simulink model "Anti_Surge_Controller_Revised"  (R2021a)
settings: Solver=VariableStepAuto  StartTime=0.0  StopTime=100  RelTol=1e-3
values from neighbouring files (symbols this model uses):
  AolT = sys_dt.A    [zhu_model_magnetic_bearing.m]
  BolT = sys_dt.B    [zhu_model_magnetic_bearing.m]
  c = c1+c2+c3+c4+c5+c6    [zhu_model_magnetic_bearing.m]
  ColT = sys_dt.C    [zhu_model_magnetic_bearing.m]
  DolT = sys_dt.D    [zhu_model_magnetic_bearing.m]
  k = 25    [zhu_model_magnetic_bearing.m]
  Ki = Kflux*N/Ro    [zhu_model_magnetic_bearing.m]
  Kx = Kflux^2/Ro/25000    [zhu_model_magnetic_bearing.m]
  m = 330    [zhu_model_magnetic_bearing.m]
  P0T = 10^-3    (= 0.001)    [zhu_model_magnetic_bearing.m]
  QcovT = 10^-5    (= 1e-05)    [zhu_model_magnetic_bearing.m]
  RcovT = 10^-4    (= 0.0001)    [zhu_model_magnetic_bearing.m]
  s = fotf('s')    [zhu_model_magnetic_bearing.m]
  x0T = 0    [zhu_model_magnetic_bearing.m]
undefined symbols (not defined in the file or in its folder): K1, K2, P0, Qcov, Rcov, sys_d, x0c
libraries: simulink x4, fod x2
settings Model: Creator=NATO  LastModifiedBy=macbookpro
settings SolverCC: AlgebraicLoopSolver=TrustRegion
settings DataIOCC: ReturnWorkspaceOutputs=off
settings DebuggingCC: SFMachineParentedDataDiag=warning  ArithmeticOperatorsInVariantConditions=warning
settings SFSimCC: SimUseLocalCustomCode=off  CustomCodeUndefinedFunction=UseInterfaceOnly
settings RTWCC: RTWUseLocalCustomCode=off
settings CodeAppCC: StateflowObjectComments=on

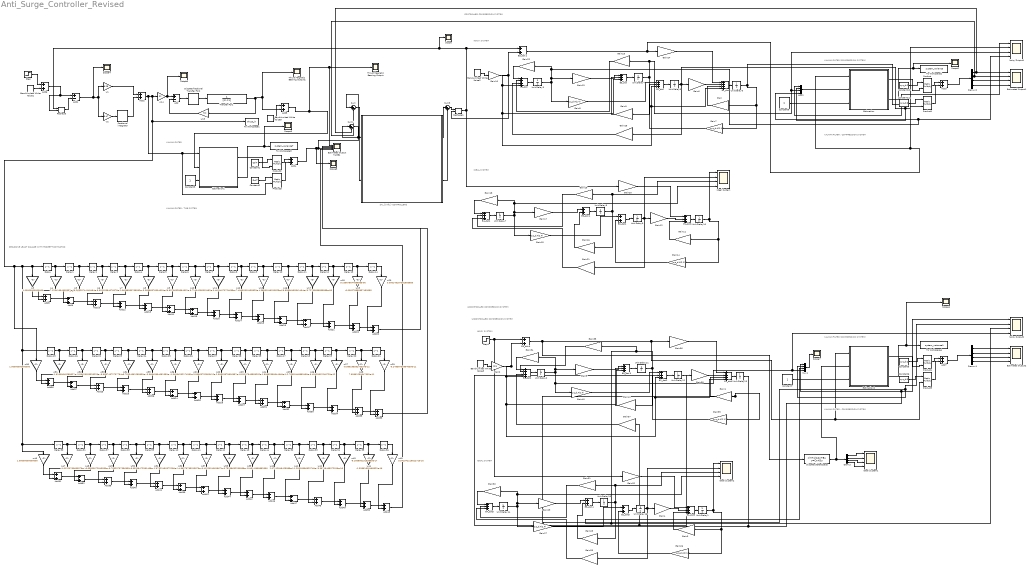
== system Anti_Surge_Controller_Revised ==
  note: RECURSIVE LEAST SQUARE WITH FORGETTING FACTOR
  note: KALMAN FILTER (COMPRESSION SYSTEM)
  note: IDEAL SYSTEM
  note: NOISY SYSTEM
  note: KALMAN FILTER
  note: NOISY SYSTEM
  note: IDEAL SYSTEM
  note: KALMAN FILTER (COMPRESSION SYSTEM)
  note: CONTROLLED COMPRESSION SYSTEM
  note: UNCONTROLLED COMPRESSION SYSTEM
  note: KALMAN FILTER : TMB SYSTEM
  note: KALMAN FILTER : COMPRESSION SYSTEM
  note: KALMAN FILTER : COMPRESSION SYSTEM
  note: $H_{\infty} CONTROLLER$
  note: UNCONTROLLED COMPRESSION SYSTEM
  " " : Subsystem
  Add : Sum  Inputs=+-
  Add1 : Sum  Inputs=+-
  Add{2..52} (51 alike) : Sum
  Band-Limited White Noise1 : simulink/Sources/Band-Limited White Noise  Cov=[10^-10]  Ts=1  seed=[23341]
  Band-Limited White Noise2 : simulink/Sources/Band-Limited White Noise  Cov=[1]  Ts=0.05  seed=[23341]
  Band-Limited White Noise3 : simulink/Sources/Band-Limited White Noise  Cov=[1]  Ts=0.005  seed=[23341]
  Band-Limited White Noise5 : simulink/Sources/Band-Limited White Noise  Cov=[10^-8]  Ts=0.1  seed=[23341]
  Constant1 : Constant  Value=ColT  VectorParams1D=off
  Constant10 : Constant  Value=sys_d.C  VectorParams1D=off
  Constant11 : Constant  Value=sys_d.D  VectorParams1D=off
  Constant2 : Constant  Value=DolT  VectorParams1D=off
  Constant3 : Constant  VectorParams1D=off
  Constant5 : Constant  Value=sys_d.C  VectorParams1D=off
  Constant6 : Constant  Value=sys_d.D  VectorParams1D=off
  Constant7 : Constant  VectorParams1D=off
  Constant9 : Constant  VectorParams1D=off
  Delay{,1..44} (45 alike) : Delay  DelayLength=1  InitialCondition=0
  Demux : Demux
  Demux1 : Demux
  Demux2 : Demux
  Discrete State-Space : DiscreteStateSpace  A=sys_d.A  B=sys_d.B  C=sys_d.C  D=sys_d.D  SampleTime=0.005
  Discrete fractional Transfer Fcn2 : fod/Discrete fractional Transfer Fcn  zeroPoly=53900  polePoly=53900+10432*s^0.5  freqRange=[0.001, 10000]  approxNum=5  useRef=off  dscrMethod=Matched  wc=0  ts=0.1
      settings: SourceProductName=FOMCON Toolbox
  E1_dot : Sum  Inputs=++++
  E1_dot1 : Sum  Inputs=+++
  E1_dot2 : Sum  Inputs=++++
  E1_dot3 : Sum  Inputs=+++
  E2_dot : Sum  Inputs=+++
  E2_dot1 : Sum
  E2_dot2 : Sum  Inputs=+++
  E2_dot3 : Sum
  "E3_dot " : Sum  Inputs=+++
  E3_dot {1..2,4..5} (4 alike) : Sum
  E3_dot 3 : Sum  Inputs=+++
  E4_dot : Sum  Inputs=++++
  E4_dot1 : Sum  Inputs=+++
  E4_dot2 : Sum  Inputs=++++
  E4_dot3 : Sum  Inputs=+++
  Estimated Output TAMB1 : Scope  NumInputPorts=5
  Estimated Output1 : Scope  NumInputPorts=4
  Estimated Output2 : Scope  NumInputPorts=4
  Estimation : Subsystem
  Estimation1 : Subsystem
  Estimation2 : Subsystem
  Fractional integrator : fod/Fractional integrator  gam=0.5  ww=[0.001; 1000]  n=5  nFod=off
      settings: SourceProductName=FOMCON Toolbox
  Gain{,1,3,11} (4 alike) : Gain  Gain=sys_d.A(1,1)
  Gain10 : Gain  Gain=0.00001
  Gain{4,6,12,38} (4 alike) : Gain  Gain=sys_d.A(1,2)
  Gain{5,13,17,19,23,29,31,35} (8 alike) : Gain  Gain=sys_d.A(3,4)
  Gain{7,14,26,39} (4 alike) : Gain  Gain=sys_d.A(2,1)
  Gain{8,15,21,25,27,33,37,40} (8 alike) : Gain  Gain=sys_d.A(2,4)
  Gain{9,16,28,41} (4 alike) : Gain  Gain=sys_d.A(3,3)
  Gain{18,22,30,34} (4 alike) : Gain  Gain=sys_d.A(4,4)
  Gain2 : Gain  Gain=0.1
  Gain{20,24,32,36} (4 alike) : Gain  Gain=sys_d.B(1,1)
  Ideal System : Scope  NumInputPorts=4
  Ideal System1 : Scope  NumInputPorts=4
  Ideal System2 : Scope  NumInputPorts=4
  Mux1 : Mux
  Mux2 : Mux
  Noisy Output1 : Scope  NumInputPorts=4
  Noisy Output2 : Scope  NumInputPorts=4
  Product{,1..5} (6 alike) : Product  Multiplication=Matrix(*)
  Reshape : Reshape  OutputDimensionality=Derive from reference input port
  Reshape1 : Reshape  OutputDimensionality=Derive from reference input port
  Scope{,1..7} (8 alike) : Scope
  Step : Step  After=1.5*10^-4  SampleTime=0
  Step1 : Step  SampleTime=0.005
  Sum : Sum  Inputs=|+-
  Sum1 : Sum  Inputs=|+-
  Sum3 : Sum  Inputs=|++
  Thrust Magnetic Bearing Output : Scope
  Thrust Magnetic Bearing Output1 : Scope
  To Workspace1 : ToWorkspace  VariableName=thrust_in  SampleTime=0.1
      settings: Save2DSignal=2-D array (concatenate along first dimension)
  To Workspace2 : ToWorkspace  VariableName=system_variance  SampleTime=-1
      settings: MaxDataPoints=1
  To Workspace3 : ToWorkspace  VariableName=system_varianceT  SampleTime=-1
      settings: MaxDataPoints=1
  To Workspace4 : ToWorkspace  VariableName=system_variance1  SampleTime=-1
      settings: MaxDataPoints=1
  Transfer Fcn1 : TransferFcn  Denominator=[m c k]
  Unit Delay{1..2,11..16} (8 alike) : UnitDelay  SampleTime=0.005  HasFrameUpgradeWarning=on
  Unit Delay{3..10} (8 alike) : UnitDelay  SampleTime=-1  HasFrameUpgradeWarning=on
  w1 : Gain  Gain=9.25
  w10 : Gain  Gain=5.71434208313482e-06
  w11 : Gain  Gain=5.44314070724695e-06
  w12 : Gain  Gain=7.49630310435823e-06
  w13 : Gain  Gain=4.36661046310525e-05
  w14 : Gain  Gain=Ki
  w15 : Gain  Gain=Kx
  w16 : Gain  Gain=8.89806493541494e-06
  w17 : Gain  Gain=5.72750856859985e-06
  w18 : Gain  Gain=9.10967864788686e-06
  w19 : Gain  Gain=-0.000278855937453055
  w2 : Gain  Gain=3.47
  w20 : Gain  Gain=0.000145187092666685
  w21 : Gain  Gain=3.05363732083412e-13
  w22 : Gain  Gain=2.90813879816957e-12
  w23 : Gain  Gain=8.81147845559202e-12
  w24 : Gain  Gain=1.80692390644948e-12
  w25 : Gain  Gain=-2.70615448883499e-11
  w26 : Gain  Gain=6.45429512248729e-12
  w27 : Gain  Gain=-5.95929555270337e-12
  w28 : Gain  Gain=7.69961250647502e-11
  w29 : Gain  Gain=-6.24538793994039e-11
  w3 : Gain  Gain=1.00000000000000
  w30 : Gain  Gain=1.00000000000000
  w31 : Gain  Gain=-1.61509045285627e-11
  w32 : Gain  Gain=3.55425153326229e-12
  w33 : Gain  Gain=-8.68574372797784e-12
  w34 : Gain  Gain=5.79134561289939e-11
  w35 : Gain  Gain=-3.96643994081353e-11
  w36 : Gain  Gain=-1.54354252174381e-12
  w37 : Gain  Gain=-3.41220240818674e-16
  w38 : Gain  Gain=5.75138632250958e-17
  w39 : Gain  Gain=10431.8999882690
  w4 : Gain  Gain=7.12541994903337e-06
  w40 : Gain  Gain=2.07112848425985e-16
  w41 : Gain  Gain=1.29318596823748e-16
  w42 : Gain  Gain=5.38716465372916e-16
  w43 : Gain  Gain=-8.16080013153855e-17
  w44 : Gain  Gain=-1.33861815468522e-16
  w45 : Gain  Gain=5.54154221662272e-16
  w46 : Gain  Gain=1.00000000000000
  w47 : Gain  Gain=-1.01120760660376e-16
  w48 : Gain  Gain=-6.63600072843550e-18
  w49 : Gain  Gain=-9.70523797356939e-16
  w5 : Gain  Gain=6.26329744149484e-06
  w50 : Gain  Gain=8.90108472381468e-17
  w51 : Gain  Gain=1.67922450372206e-16
  w52 : Gain  Gain=-4.86276795313876e-16
  w6 : Gain  Gain=5.93115384076078e-06
  w7 : Gain  Gain=2.64598950768992e-06
  w8 : Gain  Gain=5.08988376604610e-06
  w9 : Gain  Gain=6.83706528664812e-06
  wires:
  Transfer Fcn1/1 -> Thrust Magnetic Bearing Output1/1, Add5/2, w15/1
  w15/1 -> Add/2
  Add/1 -> Discrete fractional Transfer Fcn2/1
  Add1/1 -> Scope4/1, w1/1, w2/1
  w14/1 -> Scope6/1, Add/1
  Discrete fractional Transfer Fcn2/1 -> Transfer Fcn1/1
  Band-Limited White Noise5/1 -> Add5/1
  Sum/1 -> " "/2(In1)
  Demux2/1 -> Estimated Output1/1, Sum1/2
  Demux2/2 -> Estimated Output1/2, Sum/2
  w1/1 -> Add2/1
  w2/1 -> Fractional integrator/1
  Fractional integrator/1 -> Add2/2
  Add4/1 -> Scope5/1, Sum/1, Sum1/1, Estimated Output TAMB1/4  "Kalman Filter"
  Gain16/1 -> E3_dot 1/2
  Constant10/1 -> Product/1
  E4_dot/1 -> Unit Delay3/1
  Unit Delay9/1 -> Ideal System/2, Gain12/1, Gain21/1  "E2"
  Gain25/1 -> E4_dot/3
  Gain/1 -> E1_dot/3
  Gain24/1 -> E1_dot/1  "input"
  Gain13/1 -> "E3_dot "/1
  Gain8/1 -> E2_dot/1
  E2_dot/1 -> Unit Delay5/1
  Gain23/1 -> E4_dot/2
  Unit Delay5/1 -> Mux2/2, Noisy Output1/2, Gain6/1, Gain25/1  "E2"
  Gain20/1 -> E1_dot1/1  "input"
  Constant9/1 -> Estimation/3(Active)
  Unit Delay6/1 -> Gain7/1, Gain/1, Mux2/1, Noisy Output1/1  "E1"
  Product1/1 -> Add3/2
  Estimation/2(Out2) -> Scope2/1, To Workspace2/1
  Gain6/1 -> E1_dot/2
  Add3/1 -> Demux2/1
  Gain7/1 -> E2_dot/2
  Constant11/1 -> Product1/1
  E1_dot1/1 -> Unit Delay10/1
  Demux2/3 -> Estimated Output1/3
  Demux2/4 -> Estimated Output1/4
  Gain18/1 -> E4_dot1/1
  "E3_dot "/1 -> Unit Delay4/1
  Gain10/1 -> Reshape1/2, E4_dot/4, E1_dot/4, E2_dot/3, "E3_dot "/3, E3_dot 2/2
  E2_dot1/1 -> Unit Delay9/1
  Gain11/1 -> E1_dot1/3
  Gain9/1 -> "E3_dot "/2
  Unit Delay3/1 -> Gain22/1, Noisy Output1/4, Mux2/4, Gain13/1, Gain8/1  "E4"
  Mux2/1 -> Estimation/2(y[k])
  Gain17/1 -> E3_dot 1/1
  Unit Delay7/1 -> Gain18/1, Ideal System/4, Gain17/1, Gain15/1  "E4"
  Unit Delay10/1 -> Gain14/1, Gain11/1, Ideal System/1  "E1"
  Product/1 -> Add3/1
  Gain12/1 -> E1_dot1/2
  E4_dot1/1 -> Unit Delay7/1
  Estimation/1(x̂[k|k]) -> Product/2
  E1_dot/1 -> Unit Delay6/1
  Unit Delay4/1 -> Gain9/1, Gain23/1, Noisy Output1/3, Mux2/3  "E3"
  Unit Delay8/1 -> Gain16/1, Gain19/1, Ideal System/3  "E3"
  E3_dot 1/1 -> Unit Delay8/1
  Gain15/1 -> E2_dot1/1
  Gain19/1 -> E4_dot1/2
  Gain22/1 -> E4_dot/1
  Gain21/1 -> E4_dot1/3
  Gain14/1 -> E2_dot1/2
  Band-Limited White Noise2/1 -> Gain10/1
  E3_dot 2/1 -> Gain24/1, Product1/2, Estimation/1(u[k])
  Sum1/1 -> " "/1(In2)
  Reshape1/1 -> Gain20/1, Reshape/1, Scope/1, E3_dot 2/1
  Product2/1 -> Add4/1
  Constant3/1 -> Estimation1/3(Active)
  Product3/1 -> Add4/2
  Constant2/1 -> Product3/1
  Constant1/1 -> Product2/1
  Add2/1 -> Product3/2, Estimation1/1(u[k]), Delay15/1, Delay30/1, w46/1, Delay/1, w3/1, w30/1, To Workspace1/1, w14/1
  Add5/1 -> Estimation1/2(y[k]), Thrust Magnetic Bearing Output/1, Estimated Output TAMB1/1  "Real Output TMB"
  Estimation1/1(x̂[k|k]) -> Product2/2
  Estimation1/2(Out2) -> Scope3/1, To Workspace3/1
  Band-Limited White Noise1/1 -> Add6/2
  Step/1 -> Add6/1
  Constant6/1 -> Product5/1
  Gain2/1 -> E3_dot 5/2, E4_dot2/4, E1_dot2/4, E2_dot2/3, E3_dot 3/3
  Gain35/1 -> E4_dot2/2
  E3_dot 3/1 -> Unit Delay11/1
  E3_dot 5/1 -> Discrete State-Space/1, Product5/2, Estimation2/1(u[k]), Gain36/1
  E1_dot2/1 -> Unit Delay13/1
  Demux1/2 -> Estimated Output2/2
  Gain31/1 -> E4_dot3/2
  E4_dot3/1 -> Unit Delay14/1
  Constant7/1 -> Estimation2/3(Active)
  Gain36/1 -> E1_dot2/1  "input"
  Gain37/1 -> E4_dot2/3
  Gain1/1 -> E1_dot2/3
  Gain3/1 -> E1_dot3/3
  Unit Delay14/1 -> Gain30/1, Ideal System2/4, Gain29/1, Gain27/1  "E4"
  Gain4/1 -> E1_dot3/2
  E2_dot3/1 -> Unit Delay16/1
  Gain28/1 -> E3_dot 4/2
  Constant5/1 -> Product4/1
  Unit Delay16/1 -> Ideal System2/2, Gain4/1, Gain33/1  "E2"
  Demux1/4 -> Estimated Output2/4
  Gain32/1 -> E1_dot3/1  "input"
  Product4/1 -> Add7/1
  Gain40/1 -> E2_dot2/1
  E1_dot3/1 -> Unit Delay1/1
  Gain27/1 -> E2_dot3/1
  Gain38/1 -> E1_dot2/2
  Gain34/1 -> E4_dot2/1
  E3_dot 4/1 -> Unit Delay15/1
  Unit Delay12/1 -> Gain38/1, Noisy Output2/2, Mux1/2, Gain37/1  "E2"
  Unit Delay13/1 -> Gain39/1, Gain1/1, Noisy Output2/1, Mux1/1  "E1"
  Demux1/3 -> Estimated Output2/3
  Gain30/1 -> E4_dot3/1
  Product5/1 -> Add7/2
  Gain41/1 -> E3_dot 3/2
  Gain39/1 -> E2_dot2/2
  Unit Delay15/1 -> Gain28/1, Gain31/1, Ideal System2/3  "E3"
  Gain29/1 -> E3_dot 4/1
  Unit Delay2/1 -> Noisy Output2/4, Mux1/4, Gain40/1, Gain34/1, Gain5/1  "E4"
  Unit Delay11/1 -> Gain41/1, Gain35/1, Mux1/3, Noisy Output2/3  "E3"
  Unit Delay1/1 -> Gain26/1, Gain3/1, Ideal System2/1  "E1"
  E2_dot2/1 -> Unit Delay12/1
  Gain5/1 -> E3_dot 3/1
  Gain33/1 -> E4_dot3/3
  Add7/1 -> Demux1/1
  Gain26/1 -> E2_dot3/2
  Band-Limited White Noise3/1 -> Gain2/1
  Estimation2/1(x̂[k|k]) -> Product4/2
  Estimation2/2(Out2) -> Scope1/1, To Workspace4/1
  E4_dot2/1 -> Unit Delay2/1
  Demux1/1 -> Estimated Output2/1
  " "/1(Out1) -> Sum3/1
  " "/2(Out2) -> Sum3/2
  Delay1/1 -> Delay2/1, w5/1
  Delay/1 -> Delay1/1, w4/1
  w3/1 -> Add8/1
  w4/1 -> Add8/2
  Add8/1 -> Add9/1
  w5/1 -> Add9/2
  Delay2/1 -> Delay3/1, w6/1
  w6/1 -> Add10/2
  Add9/1 -> Add10/1
  Delay3/1 -> w7/1, Delay4/1
  Delay4/1 -> w8/1, Delay5/1
  Delay5/1 -> w9/1, Delay6/1
  Delay6/1 -> w10/1, Delay7/1
  Delay7/1 -> Delay8/1, w11/1
  Delay8/1 -> Delay9/1, w12/1
  Delay9/1 -> Delay10/1, w13/1
  Delay10/1 -> Delay11/1, w16/1
  Delay11/1 -> Delay12/1, w17/1
  Delay12/1 -> Delay13/1, w18/1
  Delay13/1 -> Delay14/1, w19/1
  Add13/1 -> Add11/1
  Add6/1 -> Add1/1, Reshape/2
  Add12/1 -> Add13/1
  Add15/1 -> Add16/1
  Add16/1 -> Add14/1
  Add10/1 -> Add12/1
  w7/1 -> Add12/2
  w8/1 -> Add13/2
  w9/1 -> Add11/2
  Add11/1 -> Add15/1
  w10/1 -> Add15/2
  w11/1 -> Add16/2
  Delay14/1 -> w20/1
  w12/1 -> Add14/2
  Add18/1 -> Add19/1
  w17/1 -> Add17/2
  w16/1 -> Add19/2
  Add19/1 -> Add17/1
  Add22/1 -> Add20/1
  w20/1 -> Add20/2
  w19/1 -> Add22/2
  Add21/1 -> Add22/1
  Add14/1 -> Add18/1  "RLS : Lambda =1"
  w13/1 -> Add18/2
  Add17/1 -> Add21/1  "RLS : Lambda =1"
  w18/1 -> Add21/2
  Add20/1 -> Estimated Output TAMB1/2  "RLS : Lambda =1"
  Delay16/1 -> Delay22/1, w32/1
  w36/1 -> Add24/2
  Add26/1 -> Add24/1
  w30/1 -> Add36/1
  w31/1 -> Add36/2
  Add23/1 -> Add25/1
  Add36/1 -> Add37/1
  Add28/1 -> Add29/1
  Delay15/1 -> Delay16/1, w31/1
  w26/1 -> Add30/2
  Delay22/1 -> Delay23/1, w33/1
  w25/1 -> Add32/2
  w33/1 -> Add23/2
  Delay27/1 -> Delay28/1, w22/1
  w29/1 -> Add33/2
  w35/1 -> Add26/2
  Delay23/1 -> w34/1, Delay24/1
  w32/1 -> Add37/2
  Add34/1 -> Add35/1
  Delay21/1 -> w29/1
  Delay25/1 -> w36/1, Delay26/1
  Add29/1 -> Add27/1
  Delay20/1 -> Delay21/1, w28/1
  Delay19/1 -> Delay20/1, w27/1
  Delay24/1 -> w35/1, Delay25/1
  w22/1 -> Add29/2
  w24/1 -> Add31/2
  Add25/1 -> Add26/1
  Add37/1 -> Add23/1
  w28/1 -> Add35/2
  Delay28/1 -> Delay29/1, w23/1
  Add30/1 -> Add34/1  "RLS : Lambda =1"
  w21/1 -> Add28/2
  Add27/1 -> Add31/1  "RLS : Lambda =1"
  Add32/1 -> Add30/1
  Add31/1 -> Add32/1
  w34/1 -> Add25/2
  Delay17/1 -> Delay18/1, w25/1
  Add24/1 -> Add28/1
  w27/1 -> Add34/2
  Add35/1 -> Add33/1
  Delay26/1 -> w21/1, Delay27/1
  Delay29/1 -> Delay17/1, w24/1
  w23/1 -> Add27/2
  Delay18/1 -> Delay19/1, w26/1
  Delay31/1 -> Delay37/1, w48/1
  w52/1 -> Add39/2
  Add41/1 -> Add39/1
  w46/1 -> Add51/1
  w47/1 -> Add51/2
  Add38/1 -> Add40/1
  Add51/1 -> Add52/1
  Add43/1 -> Add44/1
  Delay30/1 -> Delay31/1, w47/1
  w42/1 -> Add45/2
  Delay37/1 -> Delay38/1, w49/1
  w41/1 -> Add47/2
  w49/1 -> Add38/2
  Delay42/1 -> Delay43/1, w38/1
  w45/1 -> Add48/2
  w51/1 -> Add41/2
  Delay38/1 -> w50/1, Delay39/1
  w48/1 -> Add52/2
  Add49/1 -> Add50/1
  Delay36/1 -> w45/1
  Delay40/1 -> w52/1, Delay41/1
  Add44/1 -> Add42/1
  Delay35/1 -> Delay36/1, w44/1
  Delay34/1 -> Delay35/1, w43/1
  Delay39/1 -> w51/1, Delay40/1
  w38/1 -> Add44/2
  w40/1 -> Add46/2
  Add40/1 -> Add41/1
  Add52/1 -> Add38/1
  w44/1 -> Add50/2
  Delay43/1 -> Delay44/1, w39/1
  Add45/1 -> Add49/1  "RLS : Lambda =1"
  w37/1 -> Add43/2
  Add42/1 -> Add46/1  "RLS : Lambda =1"
  Add47/1 -> Add45/1
  Add46/1 -> Add47/1
  w50/1 -> Add40/2
  Delay32/1 -> Delay33/1, w41/1
  Add39/1 -> Add43/1
  w43/1 -> Add49/2
  Add50/1 -> Add48/1
  Delay41/1 -> w37/1, Delay42/1
  Delay44/1 -> Delay32/1, w40/1
  w39/1 -> Add42/2
  Delay33/1 -> Delay34/1, w42/1
  Add33/1 -> Estimated Output TAMB1/3  "RLS : Lambda =0.975"
  Add48/1 -> Estimated Output TAMB1/5  "RLS : Lambda =0.95"
  Step1/1 -> E3_dot 5/1, Gain32/1
  Discrete State-Space/1 -> Estimation2/2(y[k]), Demux/1
  Demux/1 -> Ideal System1/1
  Demux/2 -> Ideal System1/2
  Demux/3 -> Ideal System1/3
  Demux/4 -> Ideal System1/4
  Reshape/1 -> Add1/2
  Sum3/1 -> Reshape1/1
  Mux1/1 -> Scope7/1

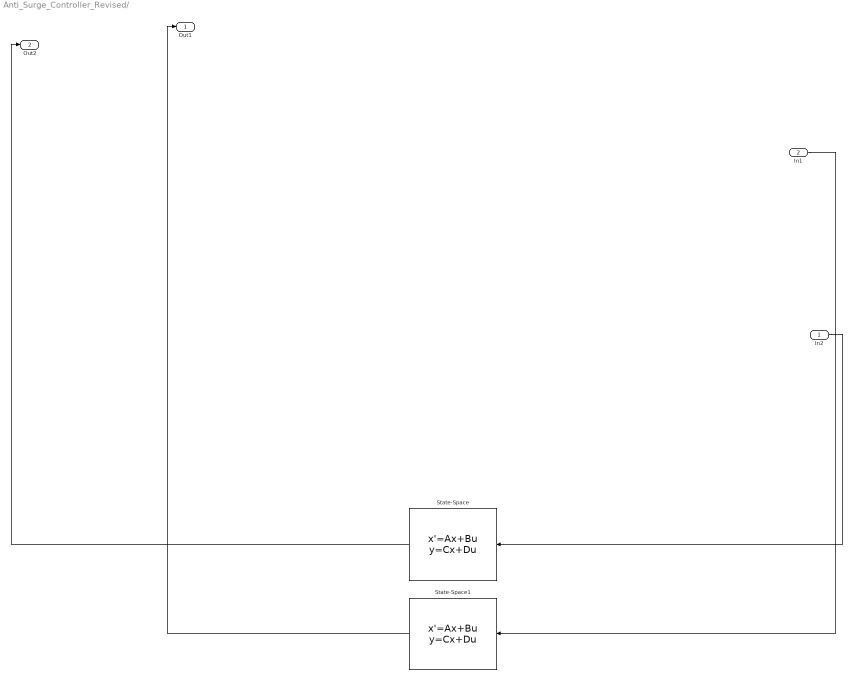
== system Anti_Surge_Controller_Revised/  ==
  In2 : Inport
  In1 : Inport  Port=2
  State-Space : StateSpace  A=K2.A  B=K2.B  C=K2.C  D=K2.D  InitialCondition=0
  State-Space1 : StateSpace  A=K1.A  B=K1.B  C=K1.C  D=K1.D  InitialCondition=0
  Out1 : Outport
  Out2 : Outport  Port=2
  wires:
  In1/1 -> State-Space1/1
  In2/1 -> State-Space/1
  State-Space1/1 -> Out1/1
  State-Space/1 -> Out2/1

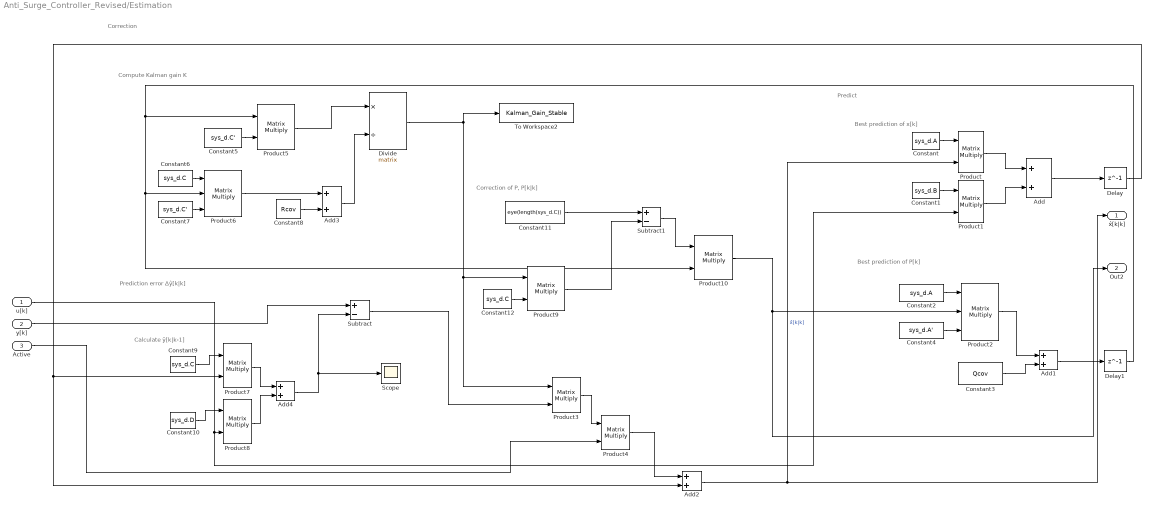
== system Anti_Surge_Controller_Revised/Estimation ==
  note: Best prediction of x[k]
  note: Predict
  note: Best prediction of P[k]
  note: Correction of P, P[k|k]
  note: Prediction error Δŷ[k|k]
  note: Compute Kalman gain K
  note: Correction
  note: Calculate ŷ[k|k-1]
  u[k] : Inport
  y[k] : Inport  Port=2
  Active : Inport  Port=3
  Add{,1..4} (5 alike) : Sum
  Constant : Constant  Value=sys_d.A  VectorParams1D=off
  Constant1 : Constant  Value=sys_d.B  VectorParams1D=off
  Constant10 : Constant  Value=sys_d.D  VectorParams1D=off
  Constant11 : Constant  Value=eye(length(sys_d.C))  VectorParams1D=off
  Constant12 : Constant  Value=sys_d.C  VectorParams1D=off
  Constant2 : Constant  Value=sys_d.A  VectorParams1D=off
  Constant3 : Constant  Value=Qcov  VectorParams1D=off
  Constant4 : Constant  Value=sys_d.A'  VectorParams1D=off
  Constant5 : Constant  Value=sys_d.C'  VectorParams1D=off
  Constant6 : Constant  Value=sys_d.C  VectorParams1D=off
  Constant7 : Constant  Value=sys_d.C'  VectorParams1D=off
  Constant8 : Constant  Value=Rcov  VectorParams1D=off
  Constant9 : Constant  Value=sys_d.C  VectorParams1D=off
  Delay : Delay  DelayLength=1  InitialCondition=x0c
  Delay1 : Delay  DelayLength=1  InitialCondition=P0
  Divide : Product  Inputs=*/  Multiplication=Matrix(*)
  Product{,1,3..5,7..10} (9 alike) : Product  Multiplication=Matrix(*)
  Product2 : Product  Inputs=3  Multiplication=Matrix(*)
  Product6 : Product  Inputs=3  Multiplication=Matrix(*)
  Scope : Scope
  Subtract : Sum  Inputs=+-
  Subtract1 : Sum  Inputs=+-
  To Workspace2 : ToWorkspace  VariableName=Kalman_Gain_Stable  SampleTime=-1
      settings: MaxDataPoints=1
  x̂[k|k] : Outport
  Out2 : Outport  Port=2
  wires:
  Constant4/1 -> Product2/3
  Constant/1 -> Product/1
  Product1/1 -> Add/2
  Constant11/1 -> Subtract1/1
  Constant6/1 -> Product6/1
  Constant12/1 -> Product9/2
  Constant2/1 -> Product2/1
  Constant3/1 -> Add1/2
  Product9/1 -> Subtract1/2
  Constant9/1 -> Product7/1
  Constant8/1 -> Add3/2
  Add3/1 -> Divide/2
  Product3/1 -> Product4/1
  u[k]/1 -> Product8/2, Product1/2
  Add/1 -> Delay/1
  Product8/1 -> Add4/2
  Add4/1 -> Subtract/2, Scope/1
  Constant5/1 -> Product5/2
  Delay/1 -> Add2/2, Product7/2
  Add2/1 -> Product/2, x̂[k|k]/1  "x̂[k|k]"
  Constant1/1 -> Product1/1
  Product/1 -> Add/1
  Active/1 -> Product4/2
  Subtract/1 -> Product3/2
  Add1/1 -> Delay1/1
  Product2/1 -> Add1/1
  Constant7/1 -> Product6/3
  Product4/1 -> Add2/1
  Delay1/1 -> Product6/2, Product10/2, Product5/1
  Product6/1 -> Add3/1
  Divide/1 -> Product3/1, Product9/1, To Workspace2/1
  y[k]/1 -> Subtract/1
  Product5/1 -> Divide/1
  Constant10/1 -> Product8/1
  Product7/1 -> Add4/1
  Product10/1 -> Out2/1, Product2/2
  Subtract1/1 -> Product10/1

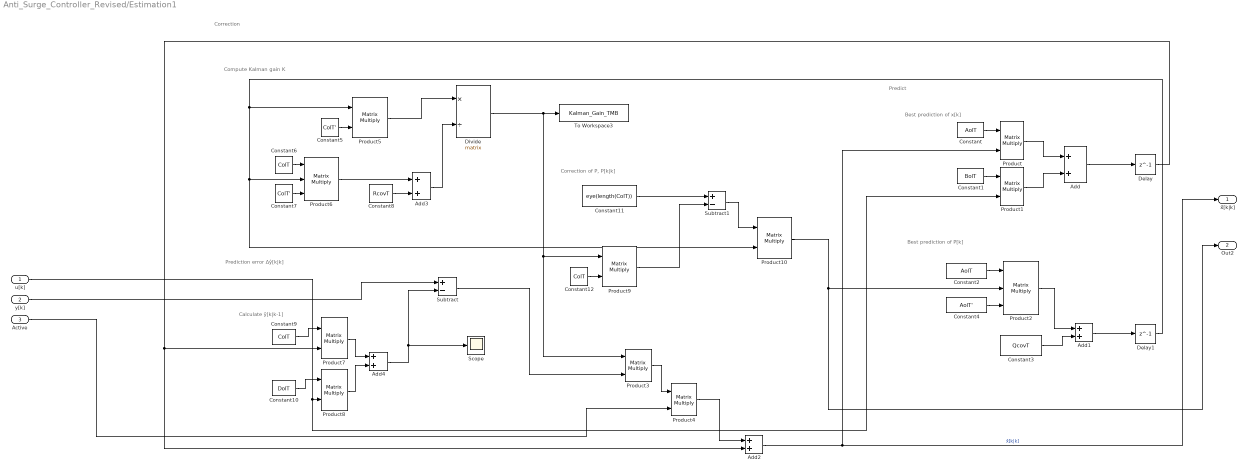
== system Anti_Surge_Controller_Revised/Estimation1 ==
  note: Best prediction of x[k]
  note: Predict
  note: Best prediction of P[k]
  note: Correction of P, P[k|k]
  note: Prediction error Δŷ[k|k]
  note: Compute Kalman gain K
  note: Correction
  note: Calculate ŷ[k|k-1]
  u[k] : Inport
  y[k] : Inport  Port=2
  Active : Inport  Port=3
  Add{,1..4} (5 alike) : Sum
  Constant : Constant  Value=AolT  VectorParams1D=off
  Constant1 : Constant  Value=BolT  VectorParams1D=off
  Constant10 : Constant  Value=DolT  VectorParams1D=off
  Constant11 : Constant  Value=eye(length(ColT))  VectorParams1D=off
  Constant12 : Constant  Value=ColT  VectorParams1D=off
  Constant2 : Constant  Value=AolT  VectorParams1D=off
  Constant3 : Constant  Value=QcovT  VectorParams1D=off
  Constant4 : Constant  Value=AolT'  VectorParams1D=off
  Constant5 : Constant  Value=ColT'  VectorParams1D=off
  Constant6 : Constant  Value=ColT  VectorParams1D=off
  Constant7 : Constant  Value=ColT'  VectorParams1D=off
  Constant8 : Constant  Value=RcovT  VectorParams1D=off
  Constant9 : Constant  Value=ColT  VectorParams1D=off
  Delay : Delay  DelayLength=1  InitialCondition=x0T
  Delay1 : Delay  DelayLength=1  InitialCondition=P0T
  Divide : Product  Inputs=*/  Multiplication=Matrix(*)
  Product{,1,3..5,7..10} (9 alike) : Product  Multiplication=Matrix(*)
  Product2 : Product  Inputs=3  Multiplication=Matrix(*)
  Product6 : Product  Inputs=3  Multiplication=Matrix(*)
  Scope : Scope
  Subtract : Sum  Inputs=+-
  Subtract1 : Sum  Inputs=+-
  To Workspace3 : ToWorkspace  VariableName=Kalman_Gain_TMB  SampleTime=-1
      settings: MaxDataPoints=1
  x̂[k|k] : Outport
  Out2 : Outport  Port=2
  wires:
  Constant4/1 -> Product2/3
  Constant/1 -> Product/1
  Product1/1 -> Add/2
  Constant11/1 -> Subtract1/1
  Constant6/1 -> Product6/1
  Constant12/1 -> Product9/2
  Constant2/1 -> Product2/1
  Constant3/1 -> Add1/2
  Product9/1 -> Subtract1/2
  Constant9/1 -> Product7/1
  Constant8/1 -> Add3/2
  Add3/1 -> Divide/2
  Product3/1 -> Product4/1
  u[k]/1 -> Product8/2, Product1/2
  Add/1 -> Delay/1
  Product8/1 -> Add4/2
  Add4/1 -> Subtract/2, Scope/1
  Constant5/1 -> Product5/2
  Delay/1 -> Add2/2, Product7/2
  Add2/1 -> Product/2, x̂[k|k]/1  "x̂[k|k]"
  Constant1/1 -> Product1/1
  Product/1 -> Add/1
  Active/1 -> Product4/2
  Subtract/1 -> Product3/2
  Add1/1 -> Delay1/1
  Product2/1 -> Add1/1
  Constant7/1 -> Product6/3
  Product4/1 -> Add2/1
  Delay1/1 -> Product6/2, Product10/2, Product5/1
  Product6/1 -> Add3/1
  Divide/1 -> Product3/1, Product9/1, To Workspace3/1
  y[k]/1 -> Subtract/1
  Product5/1 -> Divide/1
  Constant10/1 -> Product8/1
  Product7/1 -> Add4/1
  Product10/1 -> Out2/1, Product2/2
  Subtract1/1 -> Product10/1

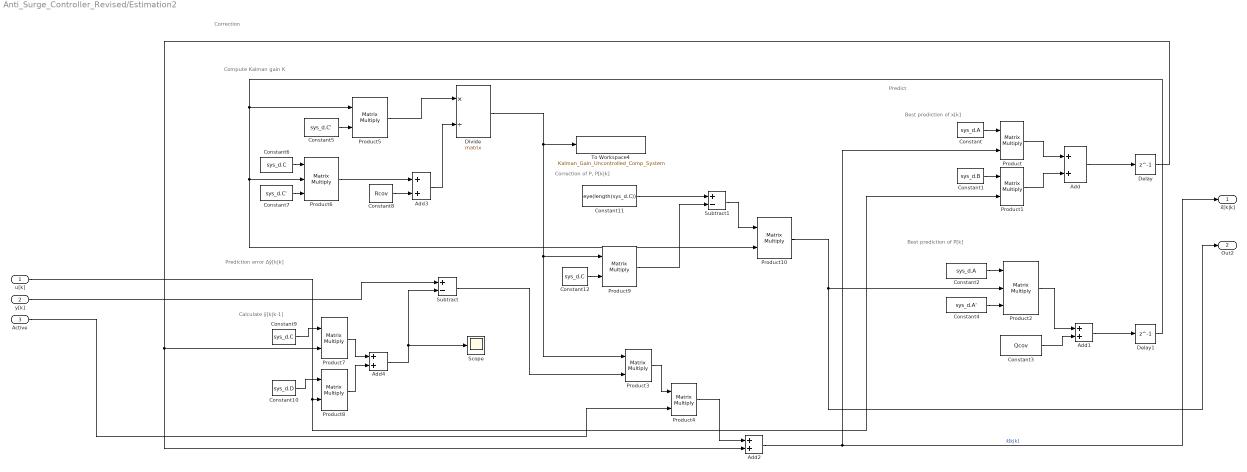
== system Anti_Surge_Controller_Revised/Estimation2 ==
  note: Best prediction of x[k]
  note: Predict
  note: Best prediction of P[k]
  note: Correction of P, P[k|k]
  note: Prediction error Δŷ[k|k]
  note: Compute Kalman gain K
  note: Correction
  note: Calculate ŷ[k|k-1]
  u[k] : Inport
  y[k] : Inport  Port=2
  Active : Inport  Port=3
  Add{,1..4} (5 alike) : Sum
  Constant : Constant  Value=sys_d.A  VectorParams1D=off
  Constant1 : Constant  Value=sys_d.B  VectorParams1D=off
  Constant10 : Constant  Value=sys_d.D  VectorParams1D=off
  Constant11 : Constant  Value=eye(length(sys_d.C))  VectorParams1D=off
  Constant12 : Constant  Value=sys_d.C  VectorParams1D=off
  Constant2 : Constant  Value=sys_d.A  VectorParams1D=off
  Constant3 : Constant  Value=Qcov  VectorParams1D=off
  Constant4 : Constant  Value=sys_d.A'  VectorParams1D=off
  Constant5 : Constant  Value=sys_d.C'  VectorParams1D=off
  Constant6 : Constant  Value=sys_d.C  VectorParams1D=off
  Constant7 : Constant  Value=sys_d.C'  VectorParams1D=off
  Constant8 : Constant  Value=Rcov  VectorParams1D=off
  Constant9 : Constant  Value=sys_d.C  VectorParams1D=off
  Delay : Delay  DelayLength=1  InitialCondition=x0c
  Delay1 : Delay  DelayLength=1  InitialCondition=P0
  Divide : Product  Inputs=*/  Multiplication=Matrix(*)
  Product{,1,3..5,7..10} (9 alike) : Product  Multiplication=Matrix(*)
  Product2 : Product  Inputs=3  Multiplication=Matrix(*)
  Product6 : Product  Inputs=3  Multiplication=Matrix(*)
  Scope : Scope
  Subtract : Sum  Inputs=+-
  Subtract1 : Sum  Inputs=+-
  To Workspace4 : ToWorkspace  VariableName=Kalman_Gain_Uncontrolled_Comp_System  SampleTime=-1
      settings: MaxDataPoints=1
  x̂[k|k] : Outport
  Out2 : Outport  Port=2
  wires:
  Constant4/1 -> Product2/3
  Constant/1 -> Product/1
  Product1/1 -> Add/2
  Constant11/1 -> Subtract1/1
  Constant6/1 -> Product6/1
  Constant12/1 -> Product9/2
  Constant2/1 -> Product2/1
  Constant3/1 -> Add1/2
  Product9/1 -> Subtract1/2
  Constant9/1 -> Product7/1
  Constant8/1 -> Add3/2
  Add3/1 -> Divide/2
  Product3/1 -> Product4/1
  u[k]/1 -> Product8/2, Product1/2
  Add/1 -> Delay/1
  Product8/1 -> Add4/2
  Add4/1 -> Subtract/2, Scope/1
  Constant5/1 -> Product5/2
  Delay/1 -> Add2/2, Product7/2
  Add2/1 -> Product/2, x̂[k|k]/1  "x̂[k|k]"
  Constant1/1 -> Product1/1
  Product/1 -> Add/1
  Active/1 -> Product4/2
  Subtract/1 -> Product3/2
  Add1/1 -> Delay1/1
  Product2/1 -> Add1/1
  Constant7/1 -> Product6/3
  Product4/1 -> Add2/1
  Delay1/1 -> Product6/2, Product10/2, Product5/1
  Product6/1 -> Add3/1
  Divide/1 -> To Workspace4/1, Product3/1, Product9/1
  y[k]/1 -> Subtract/1
  Product5/1 -> Divide/1
  Constant10/1 -> Product8/1
  Product7/1 -> Add4/1
  Product10/1 -> Out2/1, Product2/2
  Subtract1/1 -> Product10/1
